simulink model "mppt2"  (R2026a)
settings: Solver=VariableStepAuto
libraries: fl_lib x9, nesl_utility x5, ee_lib x3, batt_lib x2, batteryecm_lib x1, eePwmGenerator x1
(part 2 of 2)

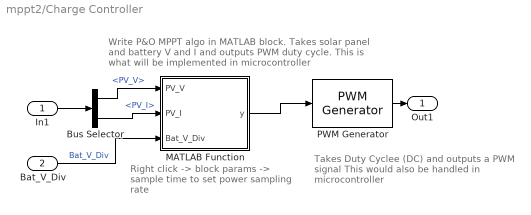
== system mppt2/Charge Controller ==
  note: Write P&O MPPT algo in MATLAB block.
      | Takes solar panel and battery V and I and outputs PWM duty cycle.
      | This is what will be implemented in microcontroller
  note: Right click -> block params -> sample time
      | to set power sampling rate
  note: Takes Duty Cyclee (DC) and outputs a PWM signal
      | This would also be handled in microcontroller
  In1 : Inport
  Bat_V_Div : Inport  Port=2
  Bus Selector : BusSelector  OutputSignals=PV_V,PV_I
  MATLAB Function : MATLAB Function  TreatAsAtomicUnit=on  SystemSampleTime=0.01
  PWM Generator : eePwmGenerator/PWM Generator  CarrCount=Up  Tper=0.001  Tdelay=0  Ts=5e-5
  Out1 : Outport
  wires:
  Bus Selector/2 -> MATLAB Function/2(PV_I)  "<PV_I>"
  MATLAB Function/1(y) -> PWM Generator/1
  In1/1 -> Bus Selector/1
  Bus Selector/1 -> MATLAB Function/1(PV_V)  "<PV_V>"
  PWM Generator/1 -> Out1/1
  Bat_V_Div/1 -> MATLAB Function/3(Bat_V_Div)  "Bat_V_Div"

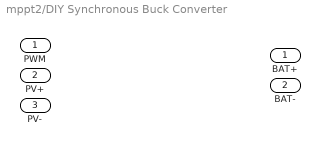
== system mppt2/DIY Synchronous Buck Converter ==
  PWM : Inport
  PV+ : Inport  Port=2
  PV- : Inport  Port=3
  BAT+ : Outport
  BAT- : Outport  Port=2

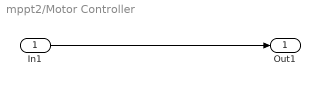
== system mppt2/Motor Controller ==
  In1 : Inport
  Out1 : Outport
  wires:
  In1/1 -> Out1/1

== matlab function mppt2/Charge Controller/MATLAB Function ==
  data: PV_V input; y output; PV_I input; Bat_V_Div input
function y = PandO(PV_V,PV_I,Bat_V_Div)
   V_Div_Ratio = 5; %Set to (Big R + Small R)/Small R of bat V divider
   Bat_V = Bat_V_Div * V_Div_Ratio; %This should recover the bat's actual V
   
 y = 1; %This will be the output(as a duty cycle)
